simulink model "simulink_bode_modified"  (R2025a)
settings: Solver=VariableStepAuto  StartTime=0.0  StopTime=10.0  RelTol=1e-3
libraries: spsSeriesRLCBranchLib x8, spsACVoltageSourceLib x1
settings Model: Creator=ASUS  LastModifiedBy=ASUS

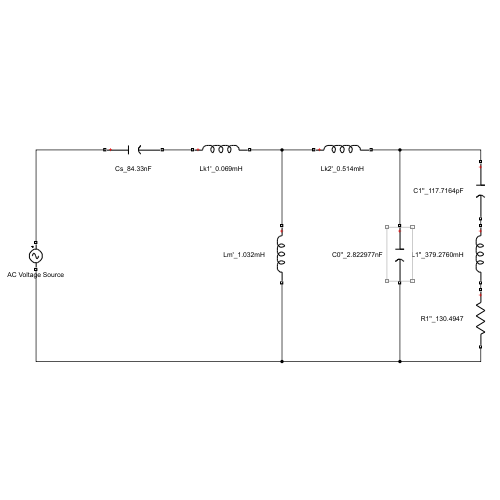
[thumbnail: Simulink's stored preview of the top-level diagram]
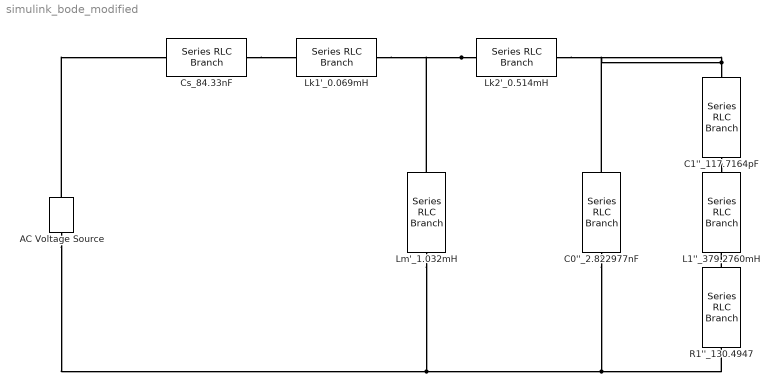
== system simulink_bode_modified ==
  AC Voltage Source : spsACVoltageSourceLib/AC Voltage Source  Amplitude=20  Phase=0  Frequency=238432  SampleTime=0  Measurements=None  BusType=swing  Pref=10e3  Qref=0  Qmin=-inf  Qmax=+inf
  C0''_2.822977nF : spsSeriesRLCBranchLib/Series RLC Branch  LConnTagsString=__new0  RConnTagsString=__new0  BranchType=C  Resistance=0  Inductance=1e-3  SetiL0=off  InitialCurrent=0  Capacitance=2.822977e-9  Setx0=off  InitialVoltage=0  Measurements=None
  C1''_117.7164pF : spsSeriesRLCBranchLib/Series RLC Branch  LConnTagsString=__new0  RConnTagsString=__new0  BranchType=C  Resistance=0  Inductance=1e-3  SetiL0=off  InitialCurrent=0  Capacitance=117.7164e-12  Setx0=off  InitialVoltage=0  Measurements=None
  Cs_84.33nF : spsSeriesRLCBranchLib/Series RLC Branch  LConnTagsString=__new0  RConnTagsString=__new0  BranchType=C  Resistance=0  Inductance=1e-3  SetiL0=off  InitialCurrent=0  Capacitance=30e-9  Setx0=off  InitialVoltage=0  Measurements=None
  L1''_379.2760mH : spsSeriesRLCBranchLib/Series RLC Branch  LConnTagsString=__new0  RConnTagsString=__new0  BranchType=L  Resistance=0  Inductance=379.2760e-3  SetiL0=off  InitialCurrent=0  Capacitance=0  Setx0=off  InitialVoltage=0  Measurements=None
  Lk1'_0.069mH : spsSeriesRLCBranchLib/Series RLC Branch  LConnTagsString=__new0  RConnTagsString=__new0  BranchType=L  Resistance=0  Inductance=0.069e-3  SetiL0=off  InitialCurrent=0  Capacitance=0  Setx0=off  InitialVoltage=0  Measurements=None
  Lk2'_0.514mH : spsSeriesRLCBranchLib/Series RLC Branch  LConnTagsString=__new0  RConnTagsString=__new0  BranchType=L  Resistance=0  Inductance=0.514e-3  SetiL0=off  InitialCurrent=0  Capacitance=0  Setx0=off  InitialVoltage=0  Measurements=None
  Lm'_1.032mH : spsSeriesRLCBranchLib/Series RLC Branch  LConnTagsString=__new0  RConnTagsString=__new0  BranchType=L  Resistance=0  Inductance=1.032e-3  SetiL0=off  InitialCurrent=0  Capacitance=0  Setx0=off  InitialVoltage=0  Measurements=None
  R1''_130.4947 : spsSeriesRLCBranchLib/Series RLC Branch  LConnTagsString=__new0  RConnTagsString=__new0  BranchType=R  Resistance=130.4947  Inductance=1e-3  SetiL0=off  InitialCurrent=0  Capacitance=0  Setx0=off  InitialVoltage=0  Measurements=None
  connections:
  C1''_117.7164pF/LConn1 -- C0''_2.822977nF/LConn1 -- Lk2'_0.514mH/RConn1
  Lk2'_0.514mH/LConn1 -- Lm'_1.032mH/LConn1 -- Lk1'_0.069mH/RConn1
  Lm'_1.032mH/RConn1 -- AC Voltage Source/LConn1 -- C0''_2.822977nF/RConn1 -- R1''_130.4947/RConn1
  Cs_84.33nF/RConn1 -- Lk1'_0.069mH/LConn1
  C1''_117.7164pF/RConn1 -- L1''_379.2760mH/LConn1
  R1''_130.4947/LConn1 -- L1''_379.2760mH/RConn1
  AC Voltage Source/RConn1 -- Cs_84.33nF/LConn1
